simulink subsystem "DCEquivalentMaxon_ECX_Flat_32L_48V_100W"  (R2026a)
settings: Solver=VariableStepAuto
libraries: ee_lib x1, fl_lib x1
settings Model: DataDictionary=neck_mk3.sldd  EnableAccessToBaseWorkspace=off  Creator=upattacini  LastModifiedBy=upattacini

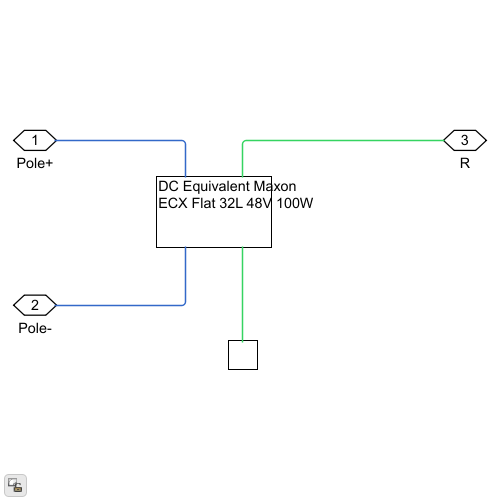
[thumbnail: Simulink's stored preview of the top-level diagram]
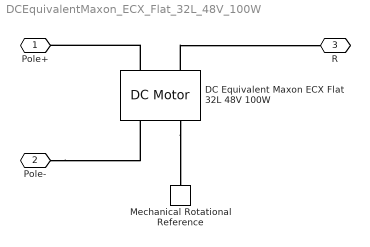
== system DCEquivalentMaxon_ECX_Flat_32L_48V_100W ==
  DC Equivalent Maxon ECX Flat 32L 48V 100W : ee_lib/Electromechanical/Brushed Motors/DC Motor  field_option=ee.enum.field_option.pm  Rf=100 Ohm  Lf=1 H  Laf=0.15 H  If0=0 A  parameterization=ee.enum.dcparam_option.circuit_param  Ra=1.07 / 2 Ohm  La=0.805 mH  emf_or_torque=ee.enum.emf_or_torque.ki  Kv=0.072e-3 V/rpm  Ki=32.8 * sqrt(3/2) mN*m/A  T_stall=0.24e-3 N*m  w_max=19100 rpm  w_rated=15000 rpm  P_rated=0.08 W  V_rated=48 V  lam_param=ee.enum.lam_param.current  i_noload=138 mA  V_i_noload=48 V  J=30.7 cm^2*g  lam=0.0010099 N*m*s/rad  speed0=0 rpm  alpha=3.93e-3 1/K  Tmeas=25 degC  thermal_mass=100 J/K  initial_temperature=25 degC
  Mechanical Rotational Reference : fl_lib/Mechanical/Rotational Elements/Mechanical Rotational Reference
  Pole+ : PMIOPort  Side=Left
  Pole- : PMIOPort  Port=2  Side=Left
  R : PMIOPort  Port=3  Side=Right
  connections:
  DC Equivalent Maxon ECX Flat 32L 48V 100W/RConn2 -- Mechanical Rotational Reference/LConn1
  DC Equivalent Maxon ECX Flat 32L 48V 100W/LConn1 -- Pole+/RConn1
  DC Equivalent Maxon ECX Flat 32L 48V 100W/LConn2 -- R/RConn1
  Pole-/RConn1 -- DC Equivalent Maxon ECX Flat 32L 48V 100W/RConn1
